simulink model "Mdl_Actuator_Test"  (R2021b)
settings: Solver=FixedStepAuto  StartTime=0.0  StopTime=10.0  FixedStep=DT  RelTol=1e-3
undefined symbols (not defined in the file): kappa, tau
settings Model: DataDictionary=DD_Mdl_Actuator.sldd  Creator=ditt_aj  LastModifiedBy=ditt_aj
settings SolverCC: AlgebraicLoopSolver=TrustRegion
settings DebuggingCC: SFMachineParentedDataDiag=warning

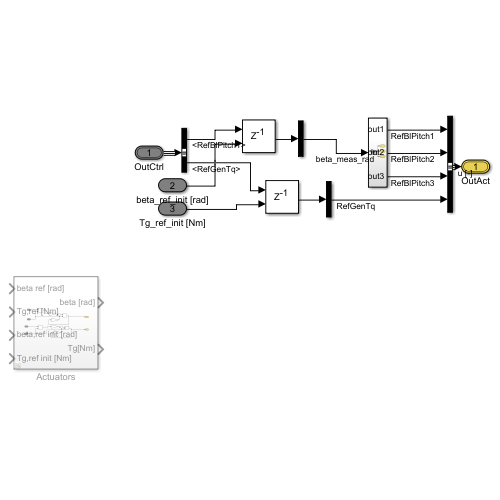
[thumbnail: Simulink's stored preview of the top-level diagram]
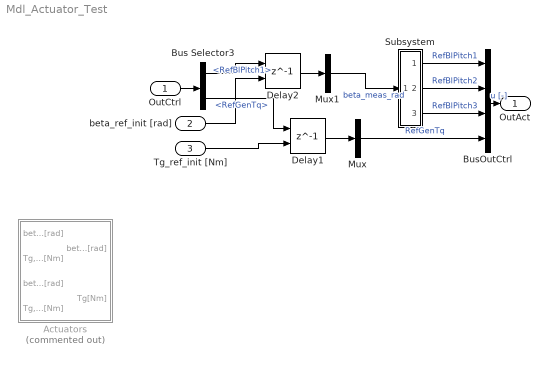
== system Mdl_Actuator_Test ==
  OutCtrl : Inport  OutDataTypeStr=Bus: slBus2
  beta_ref_init [rad] : Inport  Port=2
  Tg_ref_init [Nm] : Inport  Port=3
  Actuators : Subsystem  Commented=on
  Bus Selector3 : BusSelector  OutputSignals=RefBlPitch1,RefGenTq
  BusOutCtrl : BusCreator  Inputs=4  OutDataTypeStr=Bus: slBus2
  Delay1 : Delay  DelayLength=1  InitialConditionSource=Input port
      settings: InputPortMap=u0,p4
  Delay2 : Delay  DelayLength=1  InitialConditionSource=Input port
      settings: InputPortMap=u0,p4
  Mux : Mux  Inputs=1
  Mux1 : Mux  Inputs=1
  Subsystem : Subsystem
  OutAct : Outport  OutDataTypeStr=Bus: slBus2  VectorParamsAs1DForOutWhenUnconnected=off
  wires:
  Tg_ref_init [Nm]/1 -> Delay1/2
  beta_ref_init [rad]/1 -> Delay2/2
  OutCtrl/1 -> Bus Selector3/1
  BusOutCtrl/1 -> OutAct/1  "u [-]"
  Mux/1 -> BusOutCtrl/4  "RefGenTq"
  Mux1/1 -> Subsystem/1(in)  "beta_meas_rad"
  Subsystem/3(out3) -> BusOutCtrl/3  "RefBlPitch3"
  Subsystem/2(out2) -> BusOutCtrl/2  "RefBlPitch2"
  Subsystem/1(out1) -> BusOutCtrl/1  "RefBlPitch1"
  Delay1/1 -> Mux/1
  Bus Selector3/2 -> Delay1/1  "<RefGenTq>"
  Delay2/1 -> Mux1/1
  Bus Selector3/1 -> Delay2/1  "<RefBlPitch1>"

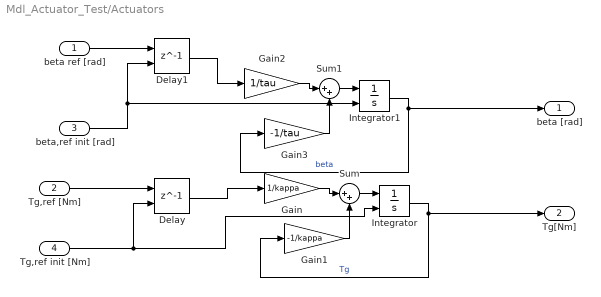
== system Mdl_Actuator_Test/Actuators ==
  beta ref [rad] : Inport
  Tg,ref [Nm] : Inport  Port=2
  beta,ref init [rad] : Inport  Port=3
  Tg,ref init [Nm] : Inport  Port=4
  Delay : Delay  DelayLength=1  InitialConditionSource=Input port
      settings: InputPortMap=u0,p4
  Delay1 : Delay  DelayLength=1  InitialConditionSource=Input port
      settings: InputPortMap=u0,p4
  Gain : Gain  Gain=1/kappa
  Gain1 : Gain  Gain=-1/kappa
  Gain2 : Gain  Gain=1/tau
  Gain3 : Gain  Gain=-1/tau
  Integrator : Integrator  InitialConditionSource=external
  Integrator1 : Integrator  InitialConditionSource=external
  Sum : Sum  Inputs=|++
  Sum1 : Sum  Inputs=|++
  beta [rad] : Outport  VectorParamsAs1DForOutWhenUnconnected=off
  Tg[Nm] : Outport  Port=2  VectorParamsAs1DForOutWhenUnconnected=off
  wires:
  Sum1/1 -> Integrator1/1
  Integrator/1 -> Tg[Nm]/1, Gain1/1  "Tg"
  Tg,ref init [Nm]/1 -> Delay/2, Integrator/2
  Gain3/1 -> Sum1/2
  Gain2/1 -> Sum1/1
  Sum/1 -> Integrator/1
  Gain1/1 -> Sum/2
  Integrator1/1 -> beta [rad]/1, Gain3/1  "beta"
  Gain/1 -> Sum/1
  Tg,ref [Nm]/1 -> Delay/1
  Delay/1 -> Gain/1
  beta ref [rad]/1 -> Delay1/1
  Delay1/1 -> Gain2/1
  beta,ref init [rad]/1 -> Integrator1/2, Delay1/2

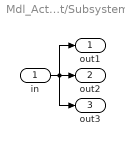
== system Mdl_Actuator_Test/Subsystem ==
  in : Inport
  out1 : Outport
  out2 : Outport  Port=2
  out3 : Outport  Port=3
  wires:
  in/1 -> out1/1, out2/1, out3/1
